simulink library "cyclopsLib"  (R2020a)
settings: Solver=VariableStepAuto  StartTime=0.0  StopTime=10.0  RelTol=1e-3
values from neighbouring files (symbols this model uses):
  agc_delay_lag = 32    [rev0BB_setup.m]
  agc_detector_coef = ones(1,agc_detector_taps)./agc_detector_taps    [rev0BB_setup.m]
  agc_sat_low = -agcSaturation    (= -12)    [rev0BB_setup.m]
  agc_sat_up = agcSaturation    (= 12)    [rev0BB_setup.m]
  agcDesired = 0    [rev0BB_setup.m]
  agcExpDomain = agcSaturation    (= 12)    [rev0BB_setup.m]
  agcExpResolution = 2^-3    (= 0.125)    [rev0BB_setup.m]
  agcPwrAvgNum = 128    [rev0BB_setup.m]
  agcSettleThresh = 0.65    [rev0BB_setup.m]
  agcStep = 2^-8    (= 0.00390625)    [rev0BB_setup.m]
  atanDomain = 5    [rev0BB_setup.m]
  atanResolution = 2^-9    (= 0.001953125)    [rev0BB_setup.m]
  bitsPerSymbolHeader = log2(radixHeader)    [rev0BB_setup.m]
  bitsPerSymbolMax = log2(radixMax)    [rev0BB_setup.m]
  cefEarlyWarning = 256    [rev0BB_setup.m]
  cefLen = length(x_CEF)    [rev0BB_setup.m]
  coarseCFOAdaptDelay = 1    [rev0BB_setup.m]
  cr_i = 0.020    (= 0.02)    [rev0BB_setup.m]
  cr_i_preamp = 2^-9    (= 0.001953125)    [rev0BB_setup.m]
  cr_int1_sat_low = -cr_integrator1_saturation    (= -0.6)    [rev0BB_setup.m]
  cr_int1_sat_up = cr_integrator1_saturation    (= 0.6)    [rev0BB_setup.m]
  cr_integrator1_decay = 1    [rev0BB_setup.m]
  cr_integrator1_saturation = 0.6    [rev0BB_setup.m]
  cr_mult_pipeline = 1    [rev0BB_setup.m]
  cr_p = 0.015    [rev0BB_setup.m]
  cr_sat2_low = -cr_saturation2    (= -0.6)    [rev0BB_setup.m]
  cr_sat2_up = cr_saturation2    (= 0.6)    [rev0BB_setup.m]
  cr_smooth_num = (1/cr_smooth_samples).*ones(1, cr_smooth_samples)    [rev0BB_setup.m]
  D_32 = [ 1,  4,  8,  2, 16]    [golay.m]    (also in rev0BB_setup.m)
  dataLenSymbols = header_len_bytes*8/bitsPerSymbolHeader + frame_len_bytes*8/bitsPerSymbol    [rev0BB_setup.m]
  delayToOutputFromDataFSM = lmsEqDepth/2-1 + regular_pipeline*9 + cr_mult_pipeline*4    (= 31)    [rev0BB_setup.m]
  enableTRFreqCorrection = true    [rev0BB_setup.m]
  expDomain = 3.3    [rev0BB_setup.m]
  expResolution = 2^-5    (= 0.03125)    [rev0BB_setup.m]
  expTol = .1    (= 0.1)    [rev0BB_setup.m]
  forceSlowRxStrobed = false    [rev0BB_setup.m]
  frac_lut_domain_cr = 64    [rev0BB_setup.m]
  frac_lut_range_max_coarse_cfo = 127    [rev0BB_setup.m]
  frac_lut_range_max_cr = 127    [rev0BB_setup.m]
  frac_lut_range_min_coarse_cfo = -frac_lut_range_max_coarse_cfo    (= -127)    [rev0BB_setup.m]
  frac_lut_range_min_cr = -frac_lut_range_max_cr    (= -127)    [rev0BB_setup.m]
  frac_lut_table_breaks_coarse_cfo = -frac_lut_domain_coarse_cfo:frac_lut_res_coarse_cfo:(frac_lut_domain_coarse_cfo-1)    [rev0BB_setup.m]
  frac_lut_table_breaks_cr = -frac_lut_domain_cr:frac_lut_res_cr:(frac_lut_domain_cr-1)    [rev0BB_setup.m]
  frac_lut_table_data_coarse_cfo = 1./frac_lut_table_breaks_coarse_cfo    [rev0BB_setup.m]
  frac_lut_table_data_cr = 1./frac_lut_table_breaks_cr    [rev0BB_setup.m]
  golay_type = 32    [rev0BB_setup.m]
  header_len_bytes = 8    [rev0BB_setup.m]
  lmsEqDepth = 38    [rev0BB_setup.m]
  lmsStep_init = 0.012    [rev0BB_setup.m]
  lmsStep_meta = (lmsStep_final - lmsStep_init)/cefLen    [rev0BB_setup.m]
  lnDomain = 16    [rev0BB_setup.m]
  lnResolution = 2^-3    (= 0.125)    [rev0BB_setup.m]
  minSTFPeaks = 3    [rev0BB_setup.m]
  mod_scheme_len_bytes = 1    [rev0BB_setup.m]
  modBPS = [1, 2, 4]    [rev0BB_setup.m]
  modKeys = [0, 1, 2]    [rev0BB_setup.m]
  mult_pipeline = 1    [rev0BB_setup.m]
  overSample = 4    [berCurve.m]    (also in rev0BB_setup.m)
  overSamplePer = 1/overSampleFreq    (= 1.25e-08)    [rev0BB_setup.m]
  qam16_demod_scale_factor = qam16_hdl_distance/qam16_power_normalized_distance    [rev0BB_setup.m]
  rcRxFilt = rcSqrtFilt    [rev0BB_setup.m]
  rcTxFilt = rcSqrtFilt    [rev0BB_setup.m]
  regular_pipeline = 1    [rev0BB_setup.m]
  rx_gain = 1    [rev0BB_setup.m]
  rx_gain_i = 1    [rev0BB_setup.m]
  rx_gain_q = 1    [rev0BB_setup.m]
  RxFeedbackPipelining = 128*3    (= 384)    [rev0BB_setup.m]
  stfLen = length(x_STF)    [rev0BB_setup.m]
  timing_differentiator_grpDelay_roundUp = ceil((timing_differentiator_len)/2)    [rev0BB_setup.m]
  timing_integrator1_decay = 0.999    [rev0BB_setup.m]
  timing_p = -1/2^2 -1/2^3    (= -0.375)    [rev0BB_setup.m]
  timing_tolerance = 4    [rev0BB_setup.m]
  timingRecoveryDoneSamplesEarly = 1    [rev0BB_setup.m]
  timingRecoveryDoneSamplesEarlyExtraDelay = -timingRecoveryDoneSamplesEarly+1    (= 0)    [rev0BB_setup.m]
  tr_int1_sat_low = -timing_integrate1_saturate    (= -0.0025)    [rev0BB_setup.m]
  tr_int1_sat_up = timing_integrate1_saturate    (= 0.0025)    [rev0BB_setup.m]
  tr_sat2_low = -timing_saturate2    (= -0.005)    [rev0BB_setup.m]
  tr_sat2_up = timing_saturate2    (= 0.005)    [rev0BB_setup.m]
  trigger = 0.40    (= 0.4)    [rev0BB_setup.m]
  trigger_tolerance = 0.35    [rev0BB_setup.m]
  W_32 = [-1,  1, -1,  1, -1]    [golay.m]    (also in rev0BB_setup.m)
  x_STFRepCount = nSpectrum_STFRepCount_short    (= 60)    [rev0BB_setup.m]
undefined symbols (not defined in the file or in its folder): agc_on, cr_integrator2_saturation, Fast_Rx_Partition, Fast_Slim_Rx_Partition, Feedback_Pipeline, freeze_en_agc, freeze_en_cr_int1, freeze_en_cr_int2, freeze_en_cr_phase, freeze_en_tr_int1, freeze_en_tr_int2, freeze_en_tr_phase, freeze_on_cef_done, freeze_on_stf_done, freeze_on_valid, i, post_cr_i_offset, post_cr_q_offset, rx_offset_correction_i, rx_offset_correction_q, Slow_Rx_Partition, timing_i, timing_i_pre_scale
libraries: simulink x62, helperLib x48, golayLib x15, commdigbbndpm3 x8, commdigbbndam3 x4, commfilt2 x3, hdlsllib x2, dspfdesign x1, simulink_need_slupdate x1, dspsigops x1, dsphdlsigops x1, $bdroot x1
(part 5 of 5)

== system cyclopsLib/cyclops_rx_combined/slow_rx_encapsulated/slow_rx/slow_rx_baseband_outer/slow_rx_baseband_enabled/slow_rx_baseband/FineCarrierRecovery/Est_Phase/atan2/bound_atan ==
  note: Bound Protection
  In1 : Inport
  Compare To Constant1 : simulink/Logic and Bit Operations/Compare To Constant  relop=>=  const=atanDomain  OutDataTypeStr=boolean
  Compare To Constant4 : simulink/Logic and Bit Operations/Compare To Constant  relop=<=  const=-atanDomain  OutDataTypeStr=boolean
  Constant11 : Constant  Value=0  OutDataTypeStr=Inherit: Inherit via back propagation  SampleTime=-1
  Constant3 : Constant  Value=pi/2  OutDataTypeStr=Inherit: Inherit via back propagation  SampleTime=-1
  Constant4 : Constant  Value=-pi/2  OutDataTypeStr=Inherit: Inherit via back propagation  SampleTime=-1
  Data Type Duplicate : DataTypeDuplicate
  Data Type Duplicate1 : DataTypeDuplicate
  Data Type Duplicate2 : DataTypeDuplicate
  Data Type Conversion : DataTypeConversion  OutDataTypeStr=single
  Logical Operator : Logic  Operator=OR  AllPortsSameDT=off  OutDataTypeStr=boolean
  Switch2 : Switch  Criteria=u2 ~= 0  OutDataTypeStr=Inherit: Inherit via back propagation
  Switch3 : Switch  Criteria=u2 ~= 0  OutDataTypeStr=Inherit: Inherit via back propagation
  Switch8 : Switch  Criteria=u2 ~= 0  OutDataTypeStr=Inherit: Inherit via back propagation
  atan Lookup Table : Lookup_n-D  NumberOfTableDimensions=1  BreakpointsForDimension1=[-atanDomain:atanResolution:atanDomain]  IndexSearchMethod=Evenly spaced points  Table=atan([-atanDomain:atanResolution:atanDomain])  InterpMethod=Flat  DiagnosticForOutOfRangeInput=Error  RemoveProtectionInput=on  InternalRulePriority=Speed  OutDataTypeStr=Inherit: Inherit via back propagation  RndMeth=Simplest  InputSameDT=on
  mult_delay : Delay  DelayLength=cr_mult_pipeline
  mult_delay_match : Delay  DelayLength=cr_mult_pipeline
  mult_delay_match1 : Delay  DelayLength=cr_mult_pipeline
  pipeline_delay1 : Delay  DelayLength=regular_pipeline*2
  pipeline_delay2 : Delay  DelayLength=regular_pipeline
  pipeline_delay_match : Delay  DelayLength=regular_pipeline*3
  pipeline_delay_match1 : Delay  DelayLength=regular_pipeline*3
  Out1 : Outport  VectorParamsAs1DForOutWhenUnconnected=off
  wires:
  pipeline_delay2/1 -> Data Type Duplicate2/1, Switch2/3
  mult_delay/1 -> atan Lookup Table/1
  pipeline_delay1/1 -> mult_delay/1
  mult_delay_match1/1 -> Switch3/2
  mult_delay_match/1 -> Switch2/2
  pipeline_delay_match1/1 -> mult_delay_match1/1
  pipeline_delay_match/1 -> mult_delay_match/1
  atan Lookup Table/1 -> Data Type Duplicate/2, pipeline_delay2/1
  Switch8/1 -> Data Type Conversion/1
  Constant11/1 -> Switch8/1
  Logical Operator/1 -> Switch8/2
  In1/1 -> Data Type Duplicate/1, Compare To Constant4/1, Compare To Constant1/1, Switch8/3
  Switch3/1 -> Data Type Duplicate2/2, Data Type Duplicate1/2, Out1/1
  Constant4/1 -> Switch3/1
  Switch2/1 -> Data Type Duplicate1/1, Switch3/3
  Constant3/1 -> Switch2/1
  Compare To Constant4/1 -> pipeline_delay_match1/1, Logical Operator/2
  Compare To Constant1/1 -> pipeline_delay_match/1, Logical Operator/1
  Data Type Conversion/1 -> pipeline_delay1/1

== system cyclopsLib/cyclops_rx_combined/slow_rx_encapsulated/slow_rx/slow_rx_baseband_outer/slow_rx_baseband_enabled/slow_rx_baseband/FineCarrierRecovery/Est_Phase/atan2/inv ==
  note: Bound Protection
  In : Inport
  Compare To Constant1 : simulink/Logic and Bit Operations/Compare To Constant  relop=>=  const=frac_lut_domain_cr-1  OutDataTypeStr=boolean
  Compare To Constant4 : simulink/Logic and Bit Operations/Compare To Constant  relop=<=  const=-frac_lut_domain_cr  OutDataTypeStr=boolean
  Constant11 : Constant  Value=0  OutDataTypeStr=Inherit: Inherit via back propagation  SampleTime=-1
  Constant3 : Constant  Value=frac_lut_range_max_cr  OutDataTypeStr=Inherit: Inherit via back propagation  SampleTime=-1
  Constant4 : Constant  Value=frac_lut_range_min_cr  OutDataTypeStr=Inherit: Inherit via back propagation  SampleTime=-1
  Data Type Duplicate : DataTypeDuplicate
  Data Type Duplicate1 : DataTypeDuplicate
  Data Type Duplicate2 : DataTypeDuplicate
  Data Type Conversion : DataTypeConversion  OutDataTypeStr=single
  Logical Operator : Logic  Operator=OR  AllPortsSameDT=off  OutDataTypeStr=boolean
  Switch2 : Switch  Criteria=u2 ~= 0  OutDataTypeStr=Inherit: Inherit via back propagation
  Switch3 : Switch  Criteria=u2 ~= 0  OutDataTypeStr=Inherit: Inherit via back propagation
  Switch8 : Switch  Criteria=u2 ~= 0  OutDataTypeStr=Inherit: Inherit via back propagation
  exp Lookup Table : Lookup_n-D  NumberOfTableDimensions=1  BreakpointsForDimension1=frac_lut_table_breaks_cr  IndexSearchMethod=Evenly spaced points  Table=frac_lut_table_data_cr  InterpMethod=Flat  DiagnosticForOutOfRangeInput=Error  RemoveProtectionInput=on  InternalRulePriority=Speed  OutDataTypeStr=Inherit: Inherit via back propagation  RndMeth=Simplest  InputSameDT=on
  mult_delay : Delay  DelayLength=cr_mult_pipeline*2
  mult_delay_match : Delay  DelayLength=cr_mult_pipeline*2
  mult_delay_match1 : Delay  DelayLength=cr_mult_pipeline*2
  pipeline_delay1 : Delay  DelayLength=regular_pipeline
  pipeline_delay2 : Delay  DelayLength=regular_pipeline  InitialCondition=1
  pipeline_delay_match : Delay  DelayLength=regular_pipeline*2
  pipeline_delay_match1 : Delay  DelayLength=regular_pipeline*2
  Out : Outport  VectorParamsAs1DForOutWhenUnconnected=off
  wires:
  pipeline_delay2/1 -> Data Type Duplicate2/1, Switch2/3
  mult_delay/1 -> exp Lookup Table/1
  pipeline_delay1/1 -> mult_delay/1
  mult_delay_match1/1 -> Switch3/2
  mult_delay_match/1 -> Switch2/2
  pipeline_delay_match1/1 -> mult_delay_match1/1
  pipeline_delay_match/1 -> mult_delay_match/1
  exp Lookup Table/1 -> Data Type Duplicate/2, pipeline_delay2/1
  Switch8/1 -> Data Type Conversion/1
  Constant11/1 -> Switch8/1
  Logical Operator/1 -> Switch8/2
  Switch3/1 -> Data Type Duplicate2/2, Data Type Duplicate1/2, Out/1
  Constant4/1 -> Switch3/1
  Switch2/1 -> Data Type Duplicate1/1, Switch3/3
  Constant3/1 -> Switch2/1
  Compare To Constant4/1 -> pipeline_delay_match1/1, Logical Operator/2
  Compare To Constant1/1 -> pipeline_delay_match/1, Logical Operator/1
  In/1 -> Data Type Duplicate/1, Compare To Constant4/1, Compare To Constant1/1, Switch8/3
  Data Type Conversion/1 -> pipeline_delay1/1

== system cyclopsLib/cyclops_rx_combined/slow_rx_encapsulated/slow_rx/slow_rx_baseband_outer/slow_rx_baseband_enabled/slow_rx_baseband/FineCarrierRecovery/scale_and_loop/Loop Filter/sat ==
  In1 : Inport
  limit_up : Inport  Port=2
  limit_low : Inport  Port=3
  Saturation : Saturate  Commented=on  UpperLimit=cr_integrator1_saturation  LowerLimit=-cr_integrator1_saturation
  Saturation Dynamic : simulink/Discontinuities/Saturation Dynamic  OutMin=[]  OutMax=[]  OutDataTypeStr=Inherit: Same as second input  OutDataType=fixdt(1, 16)  OutScaling=2^-10  DoSatur=off
  pipeline_delay : Delay  DelayLength=regular_pipeline
  Out1 : Outport  VectorParamsAs1DForOutWhenUnconnected=off
  wires:
  In1/1 -> pipeline_delay/1
  pipeline_delay/1 -> Saturation Dynamic/2
  limit_up/1 -> Saturation Dynamic/1
  limit_low/1 -> Saturation Dynamic/3
  Saturation Dynamic/1 -> Out1/1

== system cyclopsLib/cyclops_rx_combined/slow_rx_encapsulated/slow_rx/slow_rx_baseband_outer/slow_rx_baseband_enabled/slow_rx_baseband/FineCarrierRecovery/scale_and_loop/Loop Filter/sat2 ==
  In1 : Inport
  limit_up : Inport  Port=2
  limit_low : Inport  Port=3
  Saturation : Saturate  Commented=on  UpperLimit=cr_integrator2_saturation  LowerLimit=-cr_integrator2_saturation
  Saturation Dynamic : simulink/Discontinuities/Saturation Dynamic  OutMin=[]  OutMax=[]  OutDataTypeStr=Inherit: Same as second input  OutDataType=fixdt(1, 16)  OutScaling=2^-10  DoSatur=off
  pipeline_delay : Delay  DelayLength=regular_pipeline
  Out1 : Outport  VectorParamsAs1DForOutWhenUnconnected=off
  wires:
  In1/1 -> pipeline_delay/1
  limit_up/1 -> Saturation Dynamic/1
  limit_low/1 -> Saturation Dynamic/3
  pipeline_delay/1 -> Saturation Dynamic/2
  Saturation Dynamic/1 -> Out1/1

== stateflow chart cyclopsLib/cyclops_rx_combined/fast_rx/fast_rx_baseband_encapsulated/fast_rx_baseband/Timing Recovery/tr_control ==
  settings: executeAtInitialization=1
  note: Because of multipath, multiple peaks
      | may appear close together, do not
      | interpret these as error events
  state Reset
    entry:
    periodCount = int32(0);
    peakCount = int32(0);
    resetIntegerPhase=true;
    receiving=false;
    estimateOK=false;
    estimateNow=false;
    trEstDone=false;
    lastPeriod=int32(0);
  state DummyInit
    entry:
    periodCount = int32(0);
    peakCount = int32(0);
    resetIntegerPhase=true;
    receiving=false;
    estimateOK=false;
    estimateNow=false;
    trEstDone=false;
    lastPeriod=int32(0);
  state BufferFirst
    entry:
    periodCount = int32(1);
    peakCount = int32(1);
    resetIntegerPhase = true;
    receiving=true;
    estimateOK=true;
    estimateNow=true;
    trEstDone=false;
    lastPeriod=int32(golay_type*overSample);
  state WaitForNext
    entry:
    periodCount = periodCount + int32(1);
    resetIntegerPhase = false;
    receiving=true;
    estimateOK=true;
    estimateNow=false;
    trEstDone=false;
  state NextPeak
    entry:
    lastPeriod=periodCount;
    periodCount = int32(1);
    peakCount = peakCount + int32(1);
    resetIntegerPhase = false;
    receiving=true;
    estimateOK=true;
    estimateNow=true;
    trEstDone=false;
  note: Dummy initial state to ensure
      | proper init entry events occur
      | after FSM reset (from init C
      | function)
  note: This came from the packet processor in the symbol domain
  state Hold
    entry:
    resetIntegerPhase = false;
    receiving=true;
    estimateOK=false;
    estimateNow=false;
    trEstDone=true;
  (default) -> DummyInit
  Reset -> BufferFirst [order 1] : [peak == true]
  DummyInit -> Reset
  WaitForNext -> NextPeak [order 2] : [periodCount >= golay_type*(overSample-timing_tolerance) && periodCount <= golay_type*(overSample+timing_tolerance) && periodCount > overSample && peak == true]
  BufferFirst -> WaitForNext
  Reset -> Reset [order 2] : [peak == false]
  NextPeak -> WaitForNext
  WaitForNext -> Reset [order 3] : [periodCount > golay_type*(overSample+timing_tolerance)]
  WaitForNext -> WaitForNext [order 4]
  WaitForNext -> Hold [order 1] : [periodCount >= golay_type*(overSample-timing_tolerance) && periodCount <= golay_type*(overSample+timing_tolerance) && peakCount >= minSTFPeaks && peakCount <= (x_STFRepCount+1) && cef_start == true]
  Hold -> Reset : [rst == true]
  data: peak input boolean; periodCount local int32; rst input boolean; golay_type parameter int32; resetIntegerPhase output; peakCount local int32; receiving output boolean; overSample parameter int32; minSTFPeaks parameter int32; cef_start input; x_STFRepCount parameter int32; estimateOK output boolean; estimateNow output boolean; timing_tolerance parameter int32; trEstDone output boolean; lastPeriod output int32

== stateflow chart cyclopsLib/cyclops_rx_combined/slow_rx_encapsulated/slow_rx/slow_rx_baseband_outer/slow_rx_baseband_enabled/slow_rx_baseband/CoarseCFO_est/cfo_est_control ==
  settings: executeAtInitialization=1
  state Reset
    entry:
    buffer = false;
    calcDiff = false;
    periodCount = int32(0);
    peakCount = int32(0);
  state WaitForNext
    entry:
    buffer = false;
    calcDiff = false;
    periodCount = periodCount + int32(1);
  state BufferFirst
    entry:
    buffer = true;
    cur = correlation;
    calcDiff = false;
    periodCount = int32(1);
  state CalculateDiff
    entry:
    buffer = true;
    prev = cur;
    cur = correlation;
    calcDiff = true;
    peakCount = peakCount + int32(1);
    periodCount = int32(1);
  state DummyInit
    entry:
    buffer = false;
    calcDiff = false;
    periodCount = int32(0);
    peakCount = int32(0);
  note: Dummy initial state to ensure
      | proper init entry events occur
      | after FSM reset (from init C
      | function)
  state HoldDiff
    entry:
    buffer = false;
    calcDiff = false;
  CalculateDiff -> Reset [order 1] : [rst == true]
  WaitForNext -> Reset [order 1] : [rst == true]
  CalculateDiff -> WaitForNext [order 3]
  BufferFirst -> Reset [order 1] : [rst == true]
  (default) -> DummyInit
  Reset -> BufferFirst [order 1] : [peak == true]
  DummyInit -> Reset
  BufferFirst -> WaitForNext [order 3]
  WaitForNext -> CalculateDiff [order 3] : [periodCount >= golay_type ]
  Reset -> Reset [order 2] : [peak == false]
  WaitForNext -> WaitForNext [order 4]
  WaitForNext -> HoldDiff [order 2] : [stp == true]
  HoldDiff -> Reset : [rst == true]
  BufferFirst -> HoldDiff [order 2] : [stp == true]
  CalculateDiff -> HoldDiff [order 2] : [stp == true]
  data: peak input boolean; cur output; prev output; calcDiff output boolean; periodCount local int32; correlation input; stp input boolean; rst input boolean; peakCount output int32; buffer output boolean; golay_type parameter int32

== stateflow chart cyclopsLib/cyclops_rx_combined/slow_rx_encapsulated/slow_rx/slow_rx_baseband_outer/slow_rx_baseband_enabled/slow_rx_baseband/header_parse_ack_decision/header_parse_ack ==
  settings: executeAtInitialization=1
  state ParseLen
    entry:
    len = bitor(bitsrl(len, bitsPerSymbolHeader), bitsll(uint16(data), 16-bitsPerSymbolHeader));
    counter = counter + uint8(bitsPerSymbolHeader);
  state Hold
    entry:
    payload = true;
    payload_early=true;
    done_parsing = true;
  state ParseNet_Id
    entry:
    net_id = bitor(bitsrl(len, bitsPerSymbolHeader), bitsll(uint16(data), 16-bitsPerSymbolHeader));
    counter = counter + uint8(bitsPerSymbolHeader);
  state ParseDst
    entry:
    dst = bitor(bitsrl(dst, bitsPerSymbolHeader), bitsll(data, 8-bitsPerSymbolHeader));
    counter = counter + uint8(bitsPerSymbolHeader);
  state ParseSrc
    entry:
    src = bitor(bitsrl(src, bitsPerSymbolHeader), bitsll(data, 8-bitsPerSymbolHeader));
    counter = counter + uint8(bitsPerSymbolHeader);
  state ParseModType
    entry:
    mod_type = bitor(bitsrl(mod_type, bitsPerSymbolHeader),bitsll(data, 8-bitsPerSymbolHeader));
    counter = counter + uint8(bitsPerSymbolHeader);
  state Waiting
    entry:
    counter = uint8(0);
    mod_type = uint8(0);
    mod_type_valid = false;
    type = uint8(0);
    type_valid = false;
    src = uint8(0);
    src_valid = false;
    dst = uint8(0);
    dst_valid = false;
    net_id = uint16(0);
    net_id_valid = false;
    len = uint16(0);
    len_valid = false;
    done_parsing = false;
    payload = false;
    payload_early=false;
  state ParseType
    entry:
    type = bitor(bitsrl(type, bitsPerSymbolHeader),bitsll(data, 8-bitsPerSymbolHeader));
    counter = counter + uint8(bitsPerSymbolHeader);
  state DummyInit
    entry:
    counter = uint8(0);
    mod_type = uint8(0);
    mod_type_valid = false;
    type = uint8(0);
    type_valid = false;
    src = uint8(0);
    src_valid = false;
    dst = uint8(0);
    dst_valid = false;
    net_id = uint16(0);
    net_id_valid = false;
    len = uint16(0);
    len_valid = false;
    done_parsing = false;
    payload = false;
    payload_early=false;
  state ParseLenLast
    entry:
    len = bitor(bitsrl(len, bitsPerSymbolHeader), bitsll(uint16(data), 16-bitsPerSymbolHeader));
    len_valid = true;
    payload_early=true;
    counter = uint8(0);
  state ParseModTypeLast
    entry:
    mod_type = bitor(bitsrl(mod_type, bitsPerSymbolHeader), bitsll(data, 8-bitsPerSymbolHeader));
    mod_type_valid = true;
    counter = uint8(0);
  state ParseTypeLast
    entry:
    type = bitor(bitsrl(type, bitsPerSymbolHeader), bitsll(data, 8-bitsPerSymbolHeader));
    type_valid = true;
    counter = uint8(0);
  state ParseNet_IdLast
    entry:
    net_id = bitor(bitsrl(len, bitsPerSymbolHeader), bitsll(uint16(data), 16-bitsPerSymbolHeader));
    net_id_valid = true;
    counter = uint8(0);
  state ParseSrcLast
    entry:
    src = bitor(bitsrl(src, bitsPerSymbolHeader), bitsll(data, 8-bitsPerSymbolHeader));
    src_valid = true;
    counter = uint8(0);
  state ParseDstLast
    entry:
    dst = bitor(bitsrl(dst, bitsPerSymbolHeader), bitsll(data, 8-bitsPerSymbolHeader));
    dst_valid = true;
    counter = uint8(0);
  ParseLenLast -> Waiting [order 1] : [rst==true]
  ParseNet_IdLast -> Waiting [order 1] : [rst==true]
  ParseNet_Id -> Waiting [order 1] : [rst==true]
  ParseLen -> Waiting [order 1] : [rst==true]
  ParseDstLast -> Waiting [order 1] : [rst==true]
  ParseDst -> Waiting [order 1] : [rst==true]
  ParseSrcLast -> Waiting [order 1] : [rst==true]
  ParseSrc -> Waiting [order 1] : [rst==true]
  ParseTypeLast -> Waiting [order 1] : [rst==true]
  ParseType -> Waiting [order 1] : [rst==true]
  ParseModTypeLast -> Waiting [order 1] : [rst==true]
  ParseLen -> ParseLen [order 3] : [counter < 16-bitsPerSymbolHeader ]
  Hold -> Hold [order 2]
  ParseNet_Id -> ParseNet_Id [order 3] : [counter < 16-bitsPerSymbolHeader ]
  ParseModType -> Waiting [order 2] : [rst==true]
  ParseDst -> ParseDst [order 3] : [counter < 8-bitsPerSymbolHeader ]
  ParseSrc -> ParseSrc [order 3] : [counter < 8-bitsPerSymbolHeader ]
  ParseModType -> ParseModType [order 3] : [counter < 8-bitsPerSymbolHeader ]
  ParseType -> ParseType [order 3] : [counter < 8-bitsPerSymbolHeader ]
  ParseNet_IdLast -> ParseLen [order 2]
  ParseLen -> ParseLenLast [order 2] : [counter >= 16-bitsPerSymbolHeader ]
  (default) -> DummyInit
  ParseLenLast -> Hold [order 2]
  ParseDstLast -> ParseNet_Id [order 2]
  ParseNet_Id -> ParseNet_IdLast [order 2] : [counter >= 16-bitsPerSymbolHeader ]
  Waiting -> ParseModType [order 1] : [valid==true]
  Hold -> Waiting [order 1] : [rst == true]
  ParseModTypeLast -> ParseType [order 2]
  ParseType -> ParseTypeLast [order 2] : [counter >= 8-bitsPerSymbolHeader ]
  ParseModType -> ParseModTypeLast [order 1] : [counter >= 8-bitsPerSymbolHeader ]
  ParseTypeLast -> ParseSrc [order 2]
  ParseSrc -> ParseSrcLast [order 2] : [counter >= 8-bitsPerSymbolHeader ]
  ParseSrcLast -> ParseDst [order 2]
  ParseDst -> ParseDstLast [order 2] : [counter >= 8-bitsPerSymbolHeader ]
  DummyInit -> Waiting
  Waiting -> Waiting [order 2] : [valid==false]
  data: mod_type_valid output boolean; data input uint8; valid input boolean; type_valid output boolean; src_valid output boolean; dst_valid output boolean; len_valid output boolean; done_parsing output boolean; mod_type output uint8; counter local; type output uint8; src output uint8; dst output uint8; len output uint16; rst input boolean; bitsPerSymbolHeader parameter int8; payload output boolean; payload_early output boolean; net_id_valid output boolean; net_id output uint16

== stateflow chart cyclopsLib/cyclops_rx_combined/slow_rx_encapsulated/slow_rx/slow_rx_baseband_outer/slow_rx_baseband_enabled/slow_rx_baseband/mod_data_buffer/header_parse_and_buffer ==
  settings: executeAtInitialization=1
  state Exe
    note: Used if Max Modulation Scheme is BPSK
    note: Note: It is assumed that the header will exactly fit into the packed representation with no padding required. This simplifies this decoder.
    state HeaderPassThrough
      entry:
      packed_data = data;
      counter = uint8(0);
      valid = true;
      decoding=true;
    state PayloadPassThrough
      entry:
      packed_data = data;
      counter = uint8(0);
      valid = true;
    state PayloadPassThroughLast
      entry:
      packed_data = data;
      counter = uint8(0);
      valid = true;
      last_out=true;
    state FillHeaderOutput
      entry:
      packed_data = bitor(bitsrl(packed_data, bitsPerSymbolHeader),bitsll(data, bitsPerSymbolMax-bitsPerSymbolHeader));
      counter = counter + uint8(bitsPerSymbolHeader);
      valid = true;
      decoding=true;
    state FillPayloadOutput
      entry:
      packed_data = bitor(bitsrl(packed_data, bitsPerSymbolMod),bitsll(data, bitsPerSymbolMax-bitsPerSymbolMod));
      counter = counter + uint8(bitsPerSymbolMod);
      valid = true;
    state FillHeaderFirst
      entry:
      packed_data = bitsll(data, bitsPerSymbolMax-bitsPerSymbolHeader);
      counter = uint8(bitsPerSymbolHeader);
      valid = false;
    state FillHeaderMid
      entry:
      packed_data = bitor(bitsrl(packed_data, bitsPerSymbolHeader),bitsll(data, bitsPerSymbolMax-bitsPerSymbolHeader));
      counter = counter + uint8(bitsPerSymbolHeader);
      valid = false;
    state FillPayloadFirst
      entry:
      packed_data = bitsll(data, bitsPerSymbolMax-bitsPerSymbolMod);
      counter = uint8(bitsPerSymbolMod);
      valid = false;
    state FillPayloadMid
      entry:
      packed_data = bitor(bitsrl(packed_data, bitsPerSymbolMod),bitsll(data, bitsPerSymbolMax-bitsPerSymbolMod));
      counter = counter + uint8(bitsPerSymbolMod);
      valid = false;
    state FillPayloadOutputLast
      entry:
      packed_data = bitor(bitsrl(packed_data, bitsPerSymbolMod),bitsll(data, bitsPerSymbolMax-bitsPerSymbolMod));
      counter = counter + uint8(bitsPerSymbolMod);
      valid = true;
      last_out = true;
    state Err
      entry:
      last_out=true;
      err = true;
    HeaderPassThrough -> HeaderPassThrough [order 3]
    PayloadPassThrough -> PayloadPassThrough [order 2]
    HeaderPassThrough -> PayloadPassThrough [order 1] : [payload == true && bitsPerSymbolMod == bitsPerSymbolMax]
    PayloadPassThrough -> PayloadPassThroughLast [order 1] : [last_in==true]
    FillHeaderOutput -> PayloadPassThrough [order 2] : [payload == true && bitsPerSymbolMod == bitsPerSymbolMax]
    HeaderPassThrough -> FillPayloadFirst [order 2] : [payload == true && bitsPerSymbolMod ~= bitsPerSymbolMax]
    FillHeaderMid -> FillHeaderMid [order 2]
    FillPayloadMid -> FillPayloadMid [order 4]
    FillHeaderFirst -> FillHeaderMid [order 2]
    FillPayloadFirst -> FillPayloadMid [order 3]
    FillHeaderMid -> FillHeaderOutput [order 1] : [counter >=bitsPerSymbolMax-bitsPerSymbolHeader ]
    FillHeaderOutput -> FillPayloadFirst [order 1] : [payload == true && bitsPerSymbolMod ~= bitsPerSymbolMax]
    FillPayloadMid -> FillPayloadOutput [order 1] : [counter >=bitsPerSymbolMax-bitsPerSymbolMod && last_in ==false ]
    FillPayloadMid -> FillPayloadOutputLast [order 2] : [counter >=bitsPerSymbolMax-bitsPerSymbolMod && last_in ==true ]
    FillPayloadOutput -> Err [order 1] : [last_in ==true]
    FillHeaderOutput -> FillHeaderFirst [order 3]
    FillHeaderFirst -> FillHeaderOutput [order 1] : [counter >=bitsPerSymbolMax-bitsPerSymbolHeader ]
    FillPayloadFirst -> FillPayloadOutputLast [order 2] : [last_in ==true]
    FillPayloadOutput -> FillPayloadFirst [order 2]
    FillPayloadFirst -> FillPayloadOutput [order 1] : [counter >=bitsPerSymbolMax-bitsPerSymbolMod && last_in ==false ]
    FillPayloadMid -> Err [order 3] : [counter < bitsPerSymbolMax-bitsPerSymbolMod && last_in ==true ]
  state Waiting
    entry:
    counter = uint8(0);
    packed_data = uint8(0);
    valid = false;
    last_out=false;
    decoding=false;
    err=false;
  state DummyInit
    entry:
    counter = uint8(0);
    packed_data = uint8(0);
    valid = false;
    last_out=false;
    decoding=false;
    err=false;
  PayloadPassThroughLast -> Waiting
  Exe -> Waiting : [rst == true]
  Waiting -> HeaderPassThrough [order 2] : [header==true && bitsPerSymbolMax == 1]
  (default) -> DummyInit
  DummyInit -> Waiting
  Waiting -> FillHeaderFirst [order 1] : [header==true && bitsPerSymbolMax ~= 1]
  Err -> Waiting
  FillPayloadOutputLast -> Waiting
  data: last_in input boolean; header input boolean; bitsPerSymbolMax parameter uint8; bitsPerSymbolMod input uint8; last_out output boolean; packed_data output uint8; bitsPerSymbolHeader parameter uint8; data input uint8; payload input boolean; rst input boolean; valid output boolean; counter local; decoding output boolean; err output boolean

== stateflow chart cyclopsLib/cyclops_rx_combined/slow_rx_encapsulated/slow_rx/slow_rx_baseband_outer/slow_rx_baseband_enabled/slow_rx_baseband/preamble_data_ctrl/cef_eq_fsm ==
  settings: executeAtInitialization=1
  state Error
    entry:
    err = true;
    waiting = false;
  state Waiting
    entry:
    stf = false;
    cef = false;
    cef_early = false;
    data = false;
    err = false;
    ack = false;
    ack_done = false;
    ack_trigger = false;
    ack_count = uint8(0);
    ack_dst = uint8(0);
    waiting = true;
    stfCount = int32(0);
    stfPeaks = int32(0);
    cefCount = int32(0);
    cefSymb=int16(0);
  state STFFirst
    entry:
    stf = true;
    cef = false;
    cef_early = false;
    data = false;
    err = false;
    ack = false;
    ack_done = false;
    waiting = false;
    stfCount = 1;
    stfPeaks = stfPeaks + 1;
    cefSymb=int16(0);
  state STF
    entry:
    stf = true;
    cef = false;
    cef_early = false;
    data = false;
    err = false;
    ack = false;
    ack_done = false;
    waiting = false;
    stfCount = stfCount+1;
    cefSymb=int16(0);
  state DummyInit
    entry:
    stf = false;
    cef = false;
    cef_early = false;
    data = false;
    err = false;
    ack = false;
    ack_done = false;
    ack_trigger = false;
    ack_count = uint8(0);
    ack_dst = uint8(0);
    waiting = true;
    stfCount = int32(0);
    stfPeaks = int32(0);
    cefCount = int32(0);
    cefSymb=int16(0);
  state CEF_Early_Warning
    entry:
    stf = false;
    cef = true;
    cef_early = true;
    data = false;
    err = false;
    waiting = false;
    ack = false;
    ack_done = false;
    cefSymb = cefGen(cefCount+1);
    cefCount = cefCount +1;
  state LastSym
    entry:
    stf = false;
    cef = false;
    cef_early = false;
    data = true;
    err = false;
    waiting = false;
    ack = false;
    ack_done = false;
    cefSymb=int16(0);
  state CEF_Decision
    entry:
    stf = false;
    cef = true;
    cef_early = false;
    data = false;
    err = false;
    waiting = false;
    ack = false;
    ack_done = false;
    cefSymb = cefGen(cefCount+1);
    cefCount = cefCount +1;
  state CEF
    entry:
    stf = false;
    cef = true;
    cef_early = false;
    data = false;
    err = false;
    waiting = false;
    ack = false;
    ack_done = false;
    cefSymb = cefGen(cefCount+1);
    cefCount = cefCount +1;
  state Ack_First
    entry:
    stf = false;
    cef = true;
    cef_early = false;
    data = false;
    err = false;
    waiting = false;
    ack = true;
    ack_done = false;
    cefSymb = int16(0);
    cefCount = int32(1);
  state Ack_Done
    entry:
    stf = false;
    cef = false;
    cef_early = false;
    data = false;
    err = false;
    waiting = false;
    ack = true;
    ack_done = true;
    ack_trigger = false;
    cefSymb = int16(0);
    cefCount = int32(0);
  state Ack_Wait
    entry:
    stf = false;
    cef = true;
    cef_early = false;
    data = false;
    err = false;
    waiting = false;
    ack = true;
    ack_done = false;
    ack_trigger = false;
    cefSymb = int16(0);
    cefCount = cefCount +1;
  state Ack_Ca
    entry:
    stf = false;
    cef = true;
    cef_early = false;
    data = false;
    err = false;
    waiting = false;
    ack = true;
    ack_done = false;
    ack_trigger = true;
    ack_dst =  bitsrl(ack_dst, 1);
    cefSymb = int16(0);
    cefCount = int32(1);
    ack_count = ack_count + uint8(1);
  state Ack_Cb
    entry:
    stf = false;
    cef = true;
    cef_early = false;
    data = false;
    err = false;
    waiting = false;
    ack = true;
    ack_done = false;
    ack_trigger = true;
    ack_dst =  bitor(bitsrl(ack_dst, 1), bitsll(1, 7));
    cefSymb = int16(0);
    cefCount = int32(1);
    ack_count = ack_count + uint8(1);
  CEF_Decision -> Error [order 1] : [cefCount >= golay_type && ((stf_start == true && cef_start == true) || (stf_start == false && cef_start == false))]
  Ack_Wait -> Error [order 1] : [cefCount >= golay_type && ((stf_start == true && cef_start == true) || (stf_start == false && cef_start == false))]
  STF -> Error [order 1] : [stfCount >= golay_type && (stf_start==false && cef_start == false) || (stf_start==true && cef_start == true) || (cef_start == true && (stfPeaks < minSTFPeaks || stfPeaks > (x_STFRepCount+1)))]
  Error -> Waiting
  (default) -> DummyInit
  CEF_Early_Warning -> CEF_Early_Warning [order 2]
  CEF -> CEF [order 2]
  CEF_Decision -> CEF_Decision [order 4]
  STFFirst -> STF
  Waiting -> STFFirst : [stf_start==true]
  STF -> CEF_Decision [order 2] : [stfCount >= golay_type && cef_start == true && stfPeaks >= minSTFPeaks && stfPeaks <= (x_STFRepCount+1) ]
  CEF_Decision -> CEF [order 3] : [cefCount >= golay_type && stf_start == true]
  DummyInit -> Waiting
  STF -> STFFirst [order 3] : [stfCount >= golay_type && stf_start==true]
  STF -> STF [order 4]
  LastSym -> Waiting
  CEF_Early_Warning -> LastSym [order 1] : [cefCount >= cefLen]
  CEF -> CEF_Early_Warning [order 1] : [cefCount >= cefLen-cefEarlyWarning]
  CEF_Decision -> Ack_First [order 2] : [cefCount >= golay_type && cef_start == true]
  Ack_Done -> Waiting
  Ack_First -> Ack_Wait
  Ack_Wait -> Ack_Wait [order 4]
  Ack_Wait -> Ack_Cb [order 2] : [cefCount >= golay_type && stf_start == true]
  Ack_Wait -> Ack_Ca [order 3] : [cefCount >= golay_type && cef_start == true]
  Ack_Ca -> Ack_Done [order 2] : [ack_count >= 8]
  Ack_Cb -> Ack_Done [order 2] : [ack_count >= 8]
  Ack_Cb -> Ack_Wait [order 1] : [ack_count < 8]
  Ack_Ca -> Ack_Wait [order 1] : [ack_count < 8]
  data: ind function_input; symb function_output boolean; stf_start input boolean; cef_start input boolean; data output boolean; err output boolean; cefSymb output int16; stf output boolean; cef output boolean; cefCount output int32; stfCount local int32; stfLen parameter int32; cefLen parameter int32; cefEarlyWarning parameter int32; cef_early output boolean; waiting output boolean; golay_type parameter; ack_done output boolean; ack output boolean; ack_dst output uint8; ack_count output uint8; ack_trigger output boolean; x_STFRepCount parameter; minSTFPeaks parameter; stfPeaks local
  function symb = cefGen(ind):
    | function symb = cefGen(ind)
    | %128
    | % Ga_128 = [+1, +1, -1, -1, -1, -1, -1, -1, -1, +1, -1, +1, +1, -1, -1, +1, +1, +1, -1, -1, +1, +1, +1, +1, -1, +1, -1, +1, -1, +1, +1, -1, -1, -1, +1, +1, +1, +1, +1, +1, +1, -1, +1, -1, -1, +1, +1, -1, +1, +1, -1, -1, +1, +1, +1, +1, -1, +1, -1, +1, -1, +1, +1, -1, +1, +1, -1, -1, -1, -1, -1, -1, -1, +1, -1, +1, +1, -1, -1, +1, +1, +1, -1, -1, +1, +1, +1, +1, -1, +1, -1, +1, -1, +1, +1, -1, +1, +1, -1, -1, -1, -1, -1, -1, -1, +1, -1, +1, +1, -1, -1, +1, -1, -1, +1, +1, -1, -1, -1, -1, +1, -1, +1, -1, +1, -1, -1, +1];
    | % Gb_128 = [-1, -1, +1, +1, +1, +1, +1, +1, +1, -1, +1, -1, -1, +1, +1, -1, -1, -1, +1, +1, -1, -1, -1, -1, +1, -1, +1, -1, +1, -1, -1, +1, +1, +1, -1, -1, -1, -1, -1, -1, -1, +1, -1, +1, +1, -1, -1, +1, -1, -1, +1, +1, -1, -1, -1, -1, +1, -1, +1, -1, +1, -1, -1, +1, +1, +1, -1, -1, -1, -1, -1, -1, -1, +1, -1, +1, +1, -1, -1, +1, +1, +1, -1, -1, +1, +1, +1, +1, -1, +1, -1, +1, -1, +1, +1, -1, +1, +1, -1, -1, -1, -1, -1, -1, -1, +1, -1, +1, +1, -1, -1, +1, -1, -1, +1, +1, -1, -1, -1, -1, +1, -1, +1, -1, +1, -1, -1, +1];
    | % 
    | % Gu_512 = cat(2, -Gb_128, -Ga_128, Gb_128, -Ga_128);
    | % Gv_512 = cat(2, -Gb_128, Ga_128, -Gb_128, -Ga_128);
    | % Gv_128 = Gv_512(1:1:128);
    | 
    | % xSpectrum_CEF = cat(2, Gu_512, Gv_512, Gu_512, Gv_512, Gu_512, Gv_512, Gu_512, Gv_512, Gu_512, Gv_512, Gv_128);
    | % xSpectrum_CEF = cat(2, Gu_512, Gv_512, Gv_512);
    | 
    | %32
    | Ga_32  = [+1, +1, +1, +1, +1, -1, +1, -1, -1, -1, +1, +1, +1, -1, -1, +1, +1, +1, -1, -1, +1, -1, -1, +1, -1, -1, -1, -1, +1, -1, +1, -1];
    | Gb_32  = [-1, -1, -1, -1, -1, +1, -1, +1, +1, +1, -1, -1, -1, +1, +1, -1, +1, +1, -1, -1, +1, -1, -1, +1, -1, -1, -1, -1, +1, -1, +1, -1];
    | 
    | Gu_128_s = cat(2, -Gb_32, -Ga_32, Gb_32, -Ga_32);
    | Gv_128_s = cat(2, -Gb_32, Ga_32, -Gb_32, -Ga_32);
    | 
    | xSpectrum_CEF_short = cat(2, Gu_128_s, Gv_128_s, Gu_128_s, Gv_128_s, Gu_128_s, Gv_128_s, Gu_128_s, Gv_128_s, Gu_128_s, Gv_128_s, Gu_128_s, Gv_128_s, Gu_128_s, Gv_128_s);
    | %xSpectrum_CEF_short = cat(2, Gu_128_s, Gv_128_s, Gu_128_s, Gv_128_s, Gu_128_s, Gv_128_s, Gu_128_s, Gv_128_s, Gu_128_s, Gv_128_s, Gu_128_s, Gv_128_s, Gu_128_s, Gv_128_s, Gu_128_s, Gv_128_s, Gu_128_s, Gv_128_s);
    | %xSpectrum_CEF_short = cat(2, Gu_128_s, Gv_128_s, Gu_128_s, Gv_128_s, Gu_128_s, Gv_128_s, Gu_128_s, Gv_128_s, Gu_128_s, Gv_128_s, Gu_128_s, Gv_128_s, Gu_128_s, Gv_128_s, Gu_128_s, Gv_128_s, Gu_128_s, Gv_128_s, Gu_128_s, Gv_128_s, Gu_128_s, Gv_128_s, Gu_128_s, Gv_128_s, Gu_128_s, Gv_128_s, Gu_128_s, Gv_128_s);
    | 
    | 
    | symb = int16(xSpectrum_CEF_short(ind));
    | 
    | end

== stateflow chart cyclopsLib/cyclops_rx_combined/slow_rx_encapsulated/slow_rx/slow_rx_baseband_outer/slow_rx_baseband_enabled/slow_rx_baseband/preamble_data_ctrl/data_control ==
  settings: executeAtInitialization=1
  note: This is to provide a reset to the front part of the
  state Data
    entry:
    valid = true;
    last = false;
    earlyLast = false;
    dataCount = dataCount + int32(1);
  state EarlyWarningLastSym
    entry:
    valid = true;
    last = false;
    earlyLast = true;
    dataCount = dataCount + int32(1);
  state LastSym
    entry:
    valid = true;
    last = true;
    earlyLast = false;
    dataCount = dataCount + int32(1);
  state Waiting
    entry:
    valid = false;
    last = false;
    earlyLast = false;
    startCount = int32(0);
    dataCount = int32(0);
    waitCount = int32(0);
  state DummyInit
    entry:
    valid = false;
    last = false;
    startCount = int32(0);
    dataCount = int32(0);
    waitCount = int32(0);
  Data -> Data [order 2]
  EarlyWarningLastSym -> EarlyWarningLastSym [order 2]
  (default) -> DummyInit
  Waiting -> Data : [preamble_done == true]
  DummyInit -> Waiting
  LastSym -> Waiting
  Data -> EarlyWarningLastSym [order 1] : [dataCount >= dataLenSymbols-1-timingRecoveryDoneSamplesEarly]
  EarlyWarningLastSym -> LastSym [order 1] : [dataCount >= dataLenSymbols-1]
  data: preamble_done input boolean; valid output boolean; startCount local int32; dataCount local int32; waitCount local int32; dataLenSymbols parameter int32; last output boolean; earlyLast output boolean; timingRecoveryDoneSamplesEarly parameter int32
